simulink model "cambridge"  (R2023b)
settings: Solver=VariableStepAuto  StartTime=0.0  StopTime=15  FixedStep=0.0025  RelTol=1e-3
undefined symbols (not defined in the file or in its folder): body, ctrl, ground, planner, X, Y, Z
libraries: nesl_utility x71, sm_lib x43, slpidlib x24, simulink_extras x12, simulink x8, Contact_Forces_Lib x4, Parts_Lib x4, dspstat3 x1
(part 6 of 6)

== stateflow chart cambridge/Spiking neural state machine/GaitController1 ==
  settings: updateMethod=DISCRETE  sampleTime=.0025
  state superstate
    entry:
    state = 0;
    timer = 0;
    timer2 = 0;
    during:
    has_u_ctrl = [1 1 1 1];
    normal_virtual_leg1 = [0; 0; planner.stand_height];
    normal_virtual_leg2 = [0; 0; planner.stand_height];
    move_fl_end_effector = normal_virtual_leg1;
    move_rr_end_effector = normal_virtual_leg1;
    move_fr_end_effector = normal_virtual_leg2;
    move_rl_end_effector = normal_virtual_leg2;
    state Standby
      during:
      if contact_state(1) == 1 && contact_state(2) == 1 && contact_state(3) == 1 && contact_state(4) == 1
      if abs(body_vx) < planner.state0_vel_thres
      timer = timer + 1;
      else
      timer = 0;
      end
      end
    state InitSwing
      during:
      timer2 = timer2 + 1;
      % Body swing rotation
      move_theta = planner.state0_swing_ang*sin(2*pi/planner.state0_swing_T*timer2);
      move_leg_Rx = [cos(move_theta) 0 sin(move_theta);
      0 1 0;
      -sin(move_theta) 0 cos(move_theta)];
      tgt_virtual_leg1_b = move_leg_Rx*normal_virtual_leg1;
      tgt_virtual_leg2_b = move_leg_Rx*normal_virtual_leg2;
      move_fl_end_effector = tgt_virtual_leg1_b;
      move_rr_end_effector = tgt_virtual_leg1_b;
      move_fr_end_effector = tgt_virtual_leg2_b;
      move_rl_end_effector = tgt_virtual_leg2_b;
      if body_vx > planner.state12_trans_speed
      timer = timer + 1;
      else
      timer = 0;
      end
    state gait
      entry:
      % ===== SuperState: Entry =====
      % Internal state (I/O unchanged)
      hco_t = 0;  % normalized phase [0,1]
      phase_spike_count = 0;  % spikes in current phase
      spikes_per_phase = 10; % tune this for phase resolution
      during:
      % ===== SuperState: During =====
      % Assumption: spike1 and spike2 are one-tick pulses (boolean events).
      % Each event advances phase by 1/N; higher event rate => faster gait.
      if spike1 || spike2
      phase_spike_count = min(spikes_per_phase, phase_spike_count + 1);
      hco_t = phase_spike_count / spikes_per_phase;    % clamp naturally in [0,1]
      end
      state SwingLeg1
        % ===== SwingLeg1: stance VL2 (FR,RL), swing VL1 (FL,RR) =====
        % fl fr rl rr
        has_u_ctrl = [1 0 0 1];
        % Phase from spikes (implicit time via window fill)
        t = min(1.0, max(0.0, hco_t));
        % stance shaping (VL2)
        stance_length_coeff  = 0.2*t^2 - 0.2*t + 1;
        tgt_virtual_leg2_b   = stance_length_coeff * normal_virtual_leg2;
        move_fr_end_effector = tgt_virtual_leg2_b;
        move_rl_end_effector = tgt_virtual_leg2_b;
        % swing shaping (VL1)
        length_coeff = 0.6*t^2 - 0.6*t + 1;
        % fore–aft placement
        move_theta  = get_move_angle(length_coeff*normal_virtual_leg1,...
        body_vx, planner.tgt_body_vx, planner);
        move_leg_Rx = [cos(move_theta) 0  sin(move_theta);
        0              1  0;
        -sin(move_theta) 0 cos(move_theta)];
        tgt_virtual_leg1_b = length_coeff * move_leg_Rx * normal_virtual_leg1;
        % lateral / sagittal coupling
        sagittal_angle = 0.6*get_sagittal_angle(tgt_virtual_leg1_b, body_R, body_vy, planner);
        move_leg_Ry    = [1 0 0;
        0 cos(sagittal_angle) -sin(sagittal_angle);
        0 sin(sagittal_angle)  cos(sagittal_angle)];
        tgt_virtual_leg1_b = move_leg_Ry * tgt_virtual_leg1_b;
        % map to hip frames + saturation
        move_fl_end_effector = body_R'*(tgt_virtual_leg1_b + fl_offset) - fl_offset;
        if norm(move_fl_end_effector) > body.max_stretch
        move_fl_end_effector = move_fl_end_effector / norm(move_fl_end_effector) * body.max_stretch;
        end
        move_rr_end_effector = body_R'*(tgt_virtual_leg1_b + rr_offset) - rr_offset;
        if norm(move_rr_end_effector) > body.max_stretch
        move_rr_end_effector = move_rr_end_effector / norm(move_rr_end_effector) * body.max_stretch;
        end
      state SwingLeg2
        % ===== SwingLeg2: stance VL1 (FL,RR), swing VL2 (FR,RL) =====
        % fl fr rl rr
        has_u_ctrl = [0 1 1 0];
        % Phase from spikes (implicit time via window fill)
        t = min(1.0, max(0.0, hco_t));
        % stance shaping (VL1)
        stance_length_coeff  = 0.2*t^2 - 0.2*t + 1;
        tgt_virtual_leg1_b   = stance_length_coeff * normal_virtual_leg1;
        move_fl_end_effector = tgt_virtual_leg1_b;
        move_rr_end_effector = tgt_virtual_leg1_b;
        % swing shaping (VL2)
        length_coeff = 0.6*t^2 - 0.6*t + 1;
        % fore–aft placement
        move_theta  = get_move_angle(length_coeff*normal_virtual_leg2,...
        body_vx, planner.tgt_body_vx, planner);
        move_leg_Rx = [cos(move_theta) 0  sin(move_theta);
        0              1  0;
        -sin(move_theta) 0 cos(move_theta)];
        tgt_virtual_leg2_b = length_coeff * move_leg_Rx * normal_virtual_leg2;
        % lateral / sagittal coupling
        sagittal_angle = 0.6*get_sagittal_angle(tgt_virtual_leg2_b, body_R, body_vy, planner);
        move_leg_Ry    = [1 0 0;
        0 cos(sagittal_angle) -sin(sagittal_angle);
        0 sin(sagittal_angle)  cos(sagittal_angle)];
        tgt_virtual_leg2_b = move_leg_Ry * tgt_virtual_leg2_b;
        % map to hip frames + saturation
        move_fr_end_effector = body_R'*(tgt_virtual_leg2_b + fr_offset) - fr_offset;
        if norm(move_fr_end_effector) > body.max_stretch
        move_fr_end_effector = move_fr_end_effector / norm(move_fr_end_effector) * body.max_stretch;
        end
        move_rl_end_effector = body_R'*(tgt_virtual_leg2_b + rl_offset) - rl_offset;
        if norm(move_rl_end_effector) > body.max_stretch
        move_rl_end_effector = move_rl_end_effector / norm(move_rl_end_effector) * body.max_stretch;
        end
      (default) -> SwingLeg2
      SwingLeg2 -> SwingLeg1 : [ phase_spike_count >= spikes_per_phase  &&  contact_state(2)==1 && contact_state(3)==1 ]{ hco_t = 0; phase_spike_count = 0; }
      SwingLeg1 -> SwingLeg2 : [ phase_spike_count >= spikes_per_phase  &&  contact_state(1)==1 && contact_state(4)==1 ]
          | / { hco_t = 0; phase_spike_count = 0; }
    (default) -> Standby
    Standby -> InitSwing : [timer > planner.state0_trans_thres]{timer=0; state=1;}
    InitSwing -> gait : [timer>50]{timer=0; timer2=0; state=2;}
  (default) -> superstate
  data: planner parameter; body parameter; contact_state input; body_R input; body_vx input; body_vy input; fl_offset input; rl_offset input; rr_offset input; has_u_ctrl output size=[1 4] =[1 1 1 1]; move_fl_end_effector output size=[3 1] =[0;0;-0.3551]; move_fr_end_effector output size=[3 1] =[0;0;-0.3551]; move_rl_end_effector output size=[3 1] =[0;0;-0.3551]; move_rr_end_effector output size=[3 1] =[0;0;-0.3551]; state local; timer local; timer2 local; normal_virtual_leg1 local; normal_virtual_leg2 local; v2 local; Rx local; t local; t1 local; t2 local; theta local; phi local; move_theta local; Ry local; c2 local; c1 local; u1 local; u2 local; ef local; v1 local; fr_offset input; stance_length_coeff local; length_coeff local; move_leg_Ry local; sagittal_angle local; tgt_virtual_leg2_b local; move_leg_Rx local; tgt_virtual_leg1_b local; spike1 input; spike2 input; hco_t local; Ts local; t_half local; denom local; T_half_ema local; phase_flip local; phase_spike_count local; prev_spike1 local; prev_spike2 local; spk1_edge local; spikes_per_phase local; spk2_edge local

== matlab function cambridge/Spiking neural state machine/inhibitatory input1/MATLAB Function1 ==
  data: Vf input; Isyn output; Vth input; gsyn input; alpha input
function Isyn = synapse_current(Vf, Vth, gsyn, alpha)
% Current-based synapse (paper's model)
% Isyn = gsyn / (1 + exp(-alpha*(Vf - Vth)))
% Inputs:
%   Vf    - filtered presynaptic voltage (mV)
%   Vth   - threshold (mV)
%   gsyn  - synaptic strength (uA/cm^2). >0 excitatory, <0 inhibitory
%   alpha - sigmoid slope (>0)
% Output:
%   Isyn  - synaptic current to inject into postsynaptic neuron (uA/cm^2)



% Synapse nonlinearity (paper)
s = Vf - Vth;                % onto neuron 2
Isyn = gsyn / (1 + exp(-alpha * s));
end

== matlab function cambridge/Spiking neural state machine/inhibitatory input2/MATLAB Function ==
  data: Vf input; dVf output; Vi input; tau input
function dVf = synapse_filter_deriv(Vf, Vi, tau)
% ODE for the synaptic low-pass filter state Vf
% tau * dVf/dt = Vpre - Vf  ->  dVf/dt = (Vpre - Vf)/tau
% Inputs:
%   Vf   - current filter state (mV)
%   Vpre - presynaptic membrane voltage (mV)
%   tau  - filter time constant (ms, >0)
% Output:
%   dVf  - time derivative of Vf (mV/ms)

% numeric safety

dVf = 1000*(Vi - Vf) / tau;
end

== matlab function cambridge/Spiking neural state machine/inhibitatory input2/MATLAB Function1 ==
  data: Vf input; Isyn output; Vth input; gsyn input; alpha input
function Isyn = synapse_current(Vf, Vth, gsyn, alpha)
% Current-based synapse (paper's model)
% Isyn = gsyn / (1 + exp(-alpha*(Vf - Vth)))
% Inputs:
%   Vf    - filtered presynaptic voltage (mV)
%   Vth   - threshold (mV)
%   gsyn  - synaptic strength (uA/cm^2). >0 excitatory, <0 inhibitory
%   alpha - sigmoid slope (>0)
% Output:
%   Isyn  - synaptic current to inject into postsynaptic neuron (uA/cm^2)



% Synapse nonlinearity (paper)
s = Vf - Vth;                % onto neuron 2
Isyn = gsyn / (1 + exp(-alpha * s));
end

== stateflow chart cambridge/Spiking neural state machine/GaitController2 ==
  settings: updateMethod=DISCRETE  sampleTime=.0025
  state superstate
    entry:
    state = 0;
    timer = 0;
    timer2 = 0;
    during:
    has_u_ctrl = [1 1 1 1];
    normal_virtual_leg1 = [0; 0; planner.stand_height];
    normal_virtual_leg2 = [0; 0; planner.stand_height];
    move_fl_end_effector = normal_virtual_leg1;
    move_rr_end_effector = normal_virtual_leg1;
    move_fr_end_effector = normal_virtual_leg2;
    move_rl_end_effector = normal_virtual_leg2;
    state Standby
      during:
      if contact_state(1) == 1 && contact_state(2) == 1 && contact_state(3) == 1 && contact_state(4) == 1
      if abs(body_vx) < planner.state0_vel_thres
      timer = timer + 1;
      else
      timer = 0;
      end
      end
    state InitSwing
      during:
      timer2 = timer2 + 1;
      % Body swing rotation
      move_theta = planner.state0_swing_ang*sin(2*pi/planner.state0_swing_T*timer2);
      move_leg_Rx = [cos(move_theta) 0 sin(move_theta);
      0 1 0;
      -sin(move_theta) 0 cos(move_theta)];
      tgt_virtual_leg1_b = move_leg_Rx*normal_virtual_leg1;
      tgt_virtual_leg2_b = move_leg_Rx*normal_virtual_leg2;
      move_fl_end_effector = tgt_virtual_leg1_b;
      move_rr_end_effector = tgt_virtual_leg1_b;
      move_fr_end_effector = tgt_virtual_leg2_b;
      move_rl_end_effector = tgt_virtual_leg2_b;
      if body_vx > planner.state12_trans_speed
      timer = timer + 1;
      else
      timer = 0;
      end
    state gait
      state SwingLeg2
        timer2 = timer2 + 1;
        if timer2 > planner.leg_swing_time %(0.5s finish movement)
        timer2 = planner.leg_swing_time;
        end
        % stance leg no u control but need to balance the body
        % fl fr rl rr
        has_u_ctrl = [0 1 1 0];
        t = timer2/planner.leg_swing_time;
        %     stance_length_coeff = 0.95+0.05*(timer2/planner.leg_swing_time);
        stance_length_coeff = 0.2*t^2 - 0.2*t + 1;
        tgt_virtual_leg1_b = stance_length_coeff*normal_virtual_leg1;
        move_fl_end_effector = tgt_virtual_leg1_b;
        move_rr_end_effector = tgt_virtual_leg1_b;
        % swing leg must consider body angle
        %     move_theta = -11/180*pi*(t);
        length_coeff = 0.8*t^2-0.8*t+1;
        % move leg in x direction
        move_theta = get_move_angle(length_coeff*normal_virtual_leg2,body_vx, planner.tgt_body_vx, planner);
        move_leg_Rx = [cos(move_theta) 0 sin(move_theta);
        0 1 0;
        -sin(move_theta) 0 cos(move_theta)];
        tgt_virtual_leg2_b = length_coeff*move_leg_Rx*normal_virtual_leg2;
        % move leg in y direction
        sagittal_angle = get_sagittal_angle(tgt_virtual_leg2_b,body_R, body_vy, planner);
        move_leg_Ry =[1 0 0;
        0 cos(sagittal_angle) -sin(sagittal_angle);
        0 sin(sagittal_angle) cos(sagittal_angle)];
        tgt_virtual_leg2_b = move_leg_Ry*tgt_virtual_leg2_b;
        move_fr_end_effector = body_R'*(tgt_virtual_leg2_b+fr_offset)-fr_offset;
        if norm(move_fr_end_effector) > body.max_stretch
        move_fr_end_effector = move_fr_end_effector/norm(move_fr_end_effector)*body.max_stretch;
        end
        move_rl_end_effector = body_R'*(tgt_virtual_leg2_b+rl_offset)-rl_offset;
        if norm(move_rl_end_effector) > body.max_stretch
        move_rl_end_effector = move_rl_end_effector/norm(move_rl_end_effector)*body.max_stretch;
        end
        % state transition
        %     if timer2 == planner.leg_swing_time
        if timer2 > 0.5*planner.leg_swing_time && contact_state(2) == 1 && contact_state(3) == 1
        timer = timer + 1;
        else
        timer = 0;
        end
        if timer > 5   % to be determined
        state = 3;
        timer = 0;
        timer2 = 0;
        end
      state SwingLeg1
        timer2 = timer2 + 1;
        if timer2 > planner.leg_swing_time %(0.5s finish movement)
        timer2 = planner.leg_swing_time;
        end
        % stance leg no u control but need to balance the body
        % fl fr rl rr
        has_u_ctrl = [1 0 0 1];
        %     stance_length_coeff = 0.95+0.05*(timer2/planner.leg_swing_time);
        t = timer2/planner.leg_swing_time;
        stance_length_coeff = 0.2*t^2 - 0.2*t + 1;
        tgt_virtual_leg2_b = stance_length_coeff*normal_virtual_leg2;
        move_fr_end_effector = tgt_virtual_leg2_b;
        move_rl_end_effector = tgt_virtual_leg2_b;
        % swing leg must consider body angle
        % theta is a function of forward velocity
        %     move_theta = -11/180*pi*(t);
        length_coeff = 0.8*t^2-0.8*t+1;
        move_theta = get_move_angle(length_coeff*normal_virtual_leg1,body_vx, planner.tgt_body_vx, planner);
        move_leg_Rx = [cos(move_theta) 0 sin(move_theta);
        0 1 0;
        -sin(move_theta) 0 cos(move_theta)];
        tgt_virtual_leg1_b = length_coeff*move_leg_Rx*normal_virtual_leg1;
        % move leg in y direction
        sagittal_angle = get_sagittal_angle(tgt_virtual_leg1_b,body_R, body_vy, planner);
        move_leg_Ry =[1 0 0;
        0 cos(sagittal_angle) -sin(sagittal_angle);
        0 sin(sagittal_angle) cos(sagittal_angle)];
        tgt_virtual_leg1_b = move_leg_Ry*tgt_virtual_leg1_b;
        move_fl_end_effector = body_R'*(tgt_virtual_leg1_b+fl_offset)-fl_offset;
        if norm(move_fl_end_effector) > body.max_stretch
        move_fl_end_effector = move_fl_end_effector/norm(move_fl_end_effector)*body.max_stretch;
        end
        move_rr_end_effector = body_R'*(tgt_virtual_leg1_b+rr_offset)-rr_offset;
        if norm(move_rr_end_effector) > body.max_stretch
        move_rr_end_effector = move_rr_end_effector/norm(move_rr_end_effector)*body.max_stretch;
        end
        % state transition
        %     if timer2 == planner.leg_swing_time
        if timer2 > 0.5*planner.leg_swing_time && contact_state(1) == 1 && contact_state(4) == 1
        timer = timer + 1;
        else
        timer = 0;
        end
        if timer > 5   % to be determined
        state = 2;
        timer = 0;
        timer2 = 0;
        end
      (default) -> SwingLeg2
      SwingLeg2 -> SwingLeg1 : [ state==3]{timer=0; timer2=0;}
      SwingLeg1 -> SwingLeg2 : [state==2]{timer=0; timer2=0;}
    (default) -> Standby
    Standby -> InitSwing : [timer > planner.state0_trans_thres]{timer=0; state=1;}
    InitSwing -> gait : [timer>40]{timer=0; timer2=0; state=2;}
  (default) -> superstate
  data: planner parameter; body parameter; contact_state input; body_R input; body_vx input; body_vy input; fl_offset input; rl_offset input; rr_offset input; has_u_ctrl output size=[1 4] =[1 1 1 1]; move_fl_end_effector output size=[3 1] =[0;0;-0.3551]; move_fr_end_effector output size=[3 1] =[0;0;-0.3551]; move_rl_end_effector output size=[3 1] =[0;0;-0.3551]; move_rr_end_effector output size=[3 1] =[0;0;-0.3551]; state local; timer local; timer2 local; normal_virtual_leg1 local; normal_virtual_leg2 local; v2 local; Rx local; t local; t1 local; t2 local; theta local; phi local; move_theta local; Ry local; c2 local; c1 local; u1 local; u2 local; ef local; v1 local; fr_offset input; stance_length_coeff local; length_coeff local; move_leg_Ry local; sagittal_angle local; tgt_virtual_leg2_b local; move_leg_Rx local; tgt_virtual_leg1_b local; spike1 input; spike2 input

== matlab function cambridge/Spiking neural state machine/neuron1/MATLAB Function ==
  data: v input; dv output; m input; h input; n input; I_e input; dm output; dh output; dn output
function [dv, dm, dh, dn] = hh_block(v, m, h, n, I_e)
% HH ODEs for Simulink MATLAB Function block
% Inputs: v,m,h,n (states), I_e total injected current (uA/cm^2)
% Outputs: dv,dm,dh,dn (state derivatives)

    % Params
    C_m = 1.0; gNa = 120.0; gK = 36.0; gL = 0.3;
    ENa = 50.0; EK = -77.0; EL = -54.387;

    % Safe division
    am_num = 0.1 * (v + 40.0);
    am_den = 1.0 - exp(-(v + 40.0)/10.0);
    %if abs(am_den) < epsd, am_den = sign(am_den)*epsd + (am_den==0)*epsd; end
    alpha_m = am_num / am_den;

    beta_m = 4.0 * exp(-(v + 65.0)/18.0);
    alpha_h = 0.07 * exp(-(v + 65.0)/20.0);
    beta_h  = 1.0 / (1.0 + exp(-(v + 35.0)/10.0));

    an_num = 0.01 * (v + 55.0);
    an_den = 1.0 - exp(-(v + 55.0)/10.0);
    %if abs(an_den) < epsd, an_den = sign(an_den)*epsd + (an_den==0)*epsd; end
    alpha_n = an_num / an_den;

    beta_n = 0.125 * exp(-(v + 65.0)/80.0);

    % x_inf and tau
    denom_m = alpha_m + beta_m; 
    denom_h = alpha_h + beta_h; 
    denom_n = alpha_n + beta_n;

    m_inf = alpha_m / denom_m; tau_m = 1.0 / denom_m;
    h_inf = alpha_h / denom_h; tau_h = 1.0 / denom_h;
    n_inf = alpha_n / denom_n; tau_n = 1.0 / denom_n;

    % Currents
    I_Na = gNa * (m^3) * h * (v - ENa);
    I_K  = gK  * (n^4) * (v - EK);
    I_L  = gL  * (v - EL);

    % ODEs
    dv = 1000*(-I_L - I_Na - I_K + I_e) / C_m;
    dm = 1000*(m_inf - m) / tau_m;
    dh = 1000*(h_inf - h) / tau_h;
    dn = 1000*(n_inf - n) / tau_n;
end

== matlab function cambridge/Spiking neural state machine/MATLAB Function2 ==
  data: fl_ang input; eventCode output; fr_ang input; rl_ang input; rr_ang input; flags output
function [eventCode, flags] = gaitDisturbance(fl_ang, fr_ang, rl_ang, rr_ang)
% Inputs: 3x1 OR 1x3 vectors in order [shoulder; upper; knee]
% Angles can be in degrees (default) or radians—see USE_DEGREES below.
% Outputs:
%   eventCode (uint8): 0=None, 1=FL, 2=FR, 3=RL, 4=RR
%   flags (4x1 logical): [FL; FR; RL; RR] "fall down" indicators

% ---------- SETTINGS ----------
USE_DEGREES = true;     % set false if your inputs are in radians

% Nominal means and +/- bounds (DEGREES)
meansDeg  = [  0;  50; -75];   % [shoulder; upper; knee]
boundsDeg = [  10;  30;  30];  % +/- bounds

% ---------- PREP ----------
% Ensure column vectors
fl = fl_ang(:); fr = fr_ang(:); rl = rl_ang(:); rr = rr_ang(:);

% Convert to degrees if needed
if ~USE_DEGREES
    k = 180/pi;
    fl = fl.*k; fr = fr.*k; rl = rl.*k; rr = rr.*k;
end

% Compute low limits only (ignore "high" overshoot)
low  = meansDeg - boundsDeg;

% ---------- CHECK LOWER BOUNDS ONLY ----------
flFlag = any(fl < low);
frFlag = any(fr < low);
rlFlag = any(rl < low);
rrFlag = any(rr < low);
flags = logical([flFlag; frFlag; rlFlag; rrFlag]);

% Event priority: FL, FR, RL, RR
if     flFlag, eventCode = uint8(1);
elseif frFlag, eventCode = uint8(2);
elseif rlFlag, eventCode = uint8(3);
elseif rrFlag, eventCode = uint8(4);
else   eventCode = uint8(0);
end
end

== matlab function cambridge/Spiking neural state machine/neuron2/MATLAB Function ==
  data: v input; dv output; m input; h input; n input; I_e input; dm output; dh output; dn output
function [dv, dm, dh, dn] = hh_block(v, m, h, n, I_e)
% HH ODEs for Simulink MATLAB Function block
% Inputs: v,m,h,n (states), I_e total injected current (uA/cm^2)
% Outputs: dv,dm,dh,dn (state derivatives)

    % Params
    C_m = 1.0; gNa = 120.0; gK = 36.0; gL = 0.3;
    ENa = 50.0; EK = -77.0; EL = -54.387;

    % Safe division
    am_num = 0.1 * (v + 40.0);
    am_den = 1.0 - exp(-(v + 40.0)/10.0);
    %if abs(am_den) < epsd, am_den = sign(am_den)*epsd + (am_den==0)*epsd; end
    alpha_m = am_num / am_den;

    beta_m = 4.0 * exp(-(v + 65.0)/18.0);
    alpha_h = 0.07 * exp(-(v + 65.0)/20.0);
    beta_h  = 1.0 / (1.0 + exp(-(v + 35.0)/10.0));

    an_num = 0.01 * (v + 55.0);
    an_den = 1.0 - exp(-(v + 55.0)/10.0);
    %if abs(an_den) < epsd, an_den = sign(an_den)*epsd + (an_den==0)*epsd; end
    alpha_n = an_num / an_den;

    beta_n = 0.125 * exp(-(v + 65.0)/80.0);

    % x_inf and tau
    denom_m = alpha_m + beta_m; 
    denom_h = alpha_h + beta_h; 
    denom_n = alpha_n + beta_n;

    m_inf = alpha_m / denom_m; tau_m = 1.0 / denom_m;
    h_inf = alpha_h / denom_h; tau_h = 1.0 / denom_h;
    n_inf = alpha_n / denom_n; tau_n = 1.0 / denom_n;

    % Currents
    I_Na = gNa * (m^3) * h * (v - ENa);
    I_K  = gK  * (n^4) * (v - EK);
    I_L  = gL  * (v - EL);

    % ODEs
    dv = 1000*(-I_L - I_Na - I_K + I_e) / C_m;
    dm = 1000*(m_inf - m) / tau_m;
    dh = 1000*(h_inf - h) / tau_h;
    dn = 1000*(n_inf - n) / tau_n;
end
